simulink model "base_model_2021a_WS2223_controlled"  (R2021a)
settings: Solver=FixedStepDiscrete  StartTime=0.0  StopTime=10  FixedStep=0.01  RelTol=1e-3
libraries: simulink x5, pid_lib x1
settings Model: Creator=paulplusx  LastModifiedBy=erikd
settings SolverCC: AlgebraicLoopSolver=TrustRegion
settings DebuggingCC: SFMachineParentedDataDiag=warning

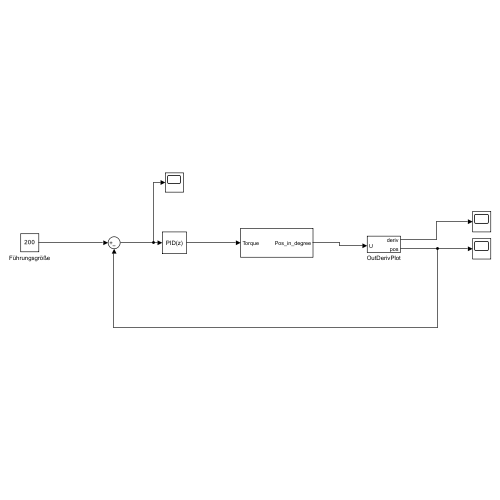
[thumbnail: Simulink's stored preview of the top-level diagram]
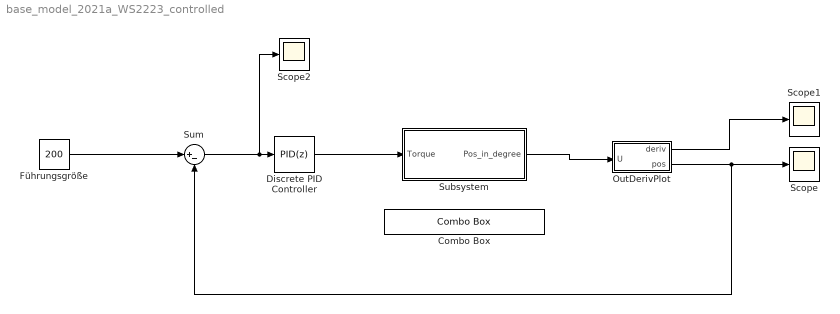
== system base_model_2021a_WS2223_controlled ==
  Combo Box : ComboBox  LabelPosition=Hide  SelectedLabel=ZERO
      settings: Values={{'ZERO', 'TYPE1', 'TYPE2', 'TYPE3', 'TYPE4', 'TYPE5', 'TYPE6', 'TYPE7', 'TYPE8', 'TYPE9'}, [0 1 2 3 4 5 6 7 8 9]}
  Discrete PID Controller : pid_lib/PID Controller  Controller=PID  Form=Parallel  TimeDomain=Discrete-time  UseExternalTs=off  SampleTime=-1  IntegratorMethod=Forward Euler  FilterMethod=Forward Euler  ControllerParametersSource=internal  P=1.02  I=0.236  D=0.059  N=100  UseFilter=on  TunerSelectOption=Transfer Function Based (PID Tuner App)  InitialConditionSource=internal  InitialConditionForIntegrator=0  InitialConditionForFilter=0  DifferentiatorICPrevScaledInput=0  ExternalReset=none  TrackingMode=off  Kt=1  LimitOutput=off  SatLimitsSource=internal  UpperSaturationLimit=inf  LowerSaturationLimit=-inf  LinearizeAsGain=off  AntiWindupMode=none  Kb=1  POutMin=[]  POutMax=[]  IOutMin=[]  IOutMax=[]  DOutMin=[]  DOutMax=[]  NOutMin=[]  NOutMax=[]  SumOutDataTypeStr=int32  SumOutMin=[]  SumOutMax=[]  SaturationOutMin=[]  SaturationOutMax=[]  PParamMin=[]  PParamMax=[]  IParamMin=[]  IParamMax=[]  DParamMin=[]  DParamMax=[]  NParamMin=[]  NParamMax=[]  KbParamMin=[]  KbParamMax=[]  KtParamMin=[]  KtParamMax=[]  KbOutMin=[]  KbOutMax=[]  KtOutMin=[]  KtOutMax=[]  IntegratorOutMin=[]  IntegratorOutMax=[]  FilterOutMin=[]  FilterOutMax=[]  SumI1OutMin=[]  SumI1OutMax=[]  SumI2OutMin=[]  SumI2OutMax=[]  SumI3OutMin=[]  SumI3OutMax=[]  SumI4OutMin=[]  SumI4OutMax=[]  SumDOutMin=[]  SumDOutMax=[]  DifferentiatorOutMin=[]  DifferentiatorOutMax=[]  FilterDiffOutCoefMin=[]  FilterDiffOutCoefMax=[]  ReciprocalOutMin=[]  ReciprocalOutMax=[]  SumDenOutMin=[]  SumDenOutMax=[]  SumNumOutMin=[]  SumNumOutMax=[]  DivideOutMin=[]  DivideOutMax=[]  UdiffTsProdOutMin=[]  UdiffTsProdOutMax=[]  NTsProdOutMin=[]  NTsProdOutMax=[]  UintegralTsProdOutMin=[]  UintegralTsProdOutMax=[]  UngainTsProdOutMin=[]  UngainTsProdOutMax=[]  IntegratorContinuousStateAttributes=''  IntegratorStateMustResolveToSignalObject=off  IntegratorRTWStateStorageClass=Auto  FilterContinuousStateAttributes=''  FilterStateMustResolveToSignalObject=off  FilterRTWStateStorageClass=Auto  ParallelPVariant=InternalParameters  IdealPVariant=Disabled  IVariant=InternalParameters  DVariant=InternalParameters  IntegratorVariant=Discrete  SatVariant=Disabled  AWVariant=Passthrough  PCopyVariant=Disabled  TRVariant=Disabled  FdbkBlocksVariant=Forward  IdealPFdbkVariant=Disabled  SatFdbkVariant=Disabled  DerivativeFilterVariant=ForwardEulerFilter  NVariant=InternalParameters  NCopyVariant=Disabled  FilterICVariant=InternalICsFilter  IntegratorICVariant=InternalICs  ExternalResetVariant=Disabled  TRSumVariant=Passthrough  SumFdbkVariant=Disabled  SumVariant=Sum_PID  TsampFilterVariant=InternalTs  TsampNgainVariant=Passthrough  TsampIntegralVariant=Passthrough  ExternalSaturationOutDataTypeStr=Inherit: Same as second input
  Führungsgröße : Constant  Value=200
  OutDerivPlot : Subsystem
  Scope : Scope
  Scope1 : Scope
  Scope2 : Scope
  Subsystem : Subsystem
  Sum : Sum  Inputs=|+-
  wires:
  Subsystem/1(Pos_in_degree) -> OutDerivPlot/1(U)
  Führungsgröße/1 -> Sum/1
  OutDerivPlot/2(pos) -> Scope/1, Sum/2
  Sum/1 -> Scope2/1, Discrete PID Controller/1
  Discrete PID Controller/1 -> Subsystem/1(Torque)
  OutDerivPlot/1(deriv) -> Scope1/1

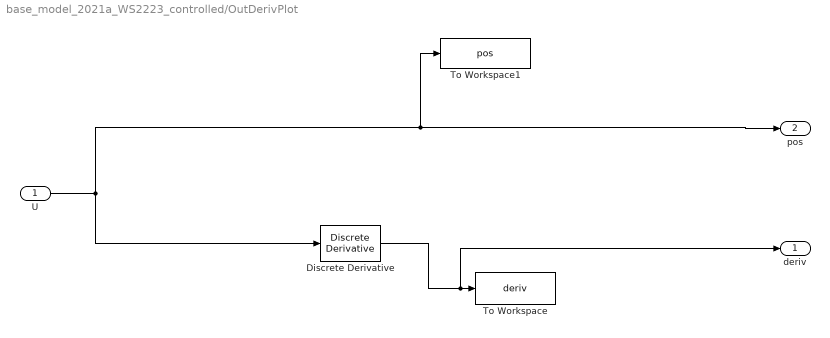
== system base_model_2021a_WS2223_controlled/OutDerivPlot ==
  U : Inport
  Discrete Derivative : simulink/Discrete/Discrete Derivative  gainval=1.0  ICPrevScaledInput=0.0  OutMin=[]  OutMax=[]  OutDataType=fixdt(1, 16)  OutScaling=2^-10  DoSatur=off
  To Workspace : ToWorkspace  VariableName=deriv  SaveFormat=Timeseries  SampleTime=-1
  To Workspace1 : ToWorkspace  VariableName=pos  SaveFormat=Timeseries  SampleTime=-1
  deriv : Outport
  pos : Outport  Port=2
  wires:
  U/1 -> pos/1, To Workspace1/1, Discrete Derivative/1
  Discrete Derivative/1 -> deriv/1, To Workspace/1

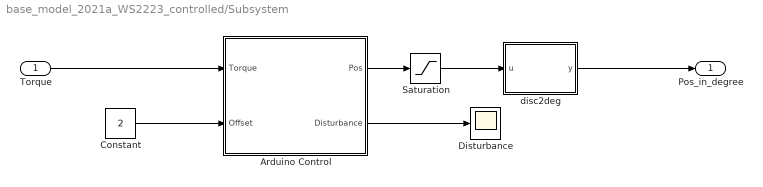
== system base_model_2021a_WS2223_controlled/Subsystem ==
  Torque : Inport
  Arduino Control : Subsystem
  Constant : Constant  Value=2  OutDataTypeStr=int32
  Disturbance : Scope
  Saturation : Saturate  UpperLimit=1024  LowerLimit=0
  disc2deg : MATLAB Function  TreatAsAtomicUnit=on
  Pos_in_degree : Outport
  wires:
  Arduino Control/1(Pos) -> Saturation/1
  Constant/1 -> Arduino Control/2(Offset)
  Arduino Control/2(Disturbance) -> Disturbance/1
  Saturation/1 -> disc2deg/1(u)
  disc2deg/1(y) -> Pos_in_degree/1
  Torque/1 -> Arduino Control/1(Torque)

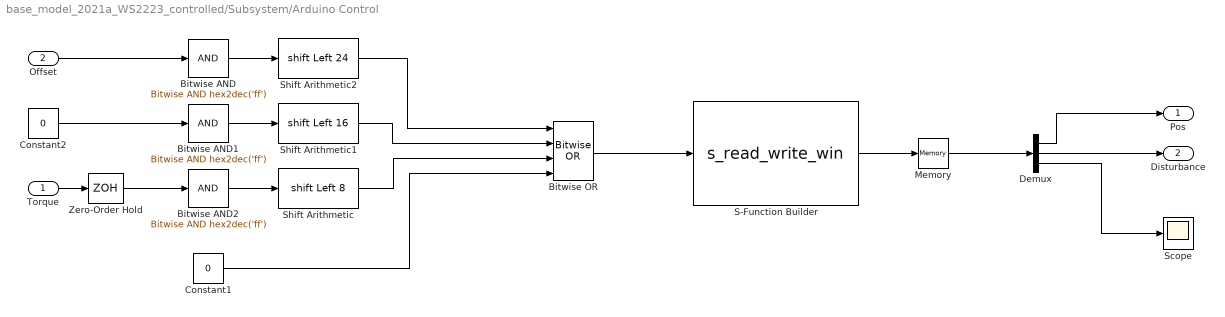
== system base_model_2021a_WS2223_controlled/Subsystem/Arduino Control ==
  Torque : Inport
  Offset : Inport  Port=2
  Bitwise AND : simulink/Logic and Bit Operations/Bitwise Operator  logicop=AND  UseBitMask=on  BitMask=hex2dec('ff')  BitMaskRealWorld=Stored Integer
  Bitwise AND1 : simulink/Logic and Bit Operations/Bitwise Operator  logicop=AND  UseBitMask=on  BitMask=hex2dec('ff')  BitMaskRealWorld=Stored Integer
  Bitwise AND2 : simulink/Logic and Bit Operations/Bitwise Operator  logicop=AND  UseBitMask=on  BitMask=hex2dec('ff')  BitMaskRealWorld=Stored Integer
  Bitwise OR : simulink/Logic and Bit Operations/Bitwise Operator  logicop=OR  UseBitMask=off  NumInputPorts=4  BitMask=bin2dec('11011001')  BitMaskRealWorld=Stored Integer
  Constant1 : Constant  Value=0  OutDataTypeStr=int32  SampleTime=-1
  Constant2 : Constant  Value=0  OutDataTypeStr=int32  SampleTime=-1
  Demux : Demux  Outputs=3
  Memory : Memory
  S-Function Builder : S-Function  FunctionName=s_read_write_win  SFunctionModules=s_read_write_win_wrapper  SFunctionDeploymentMode=off  EnableBusSupport=off  mask(S-Function Builder){}
      mask help: Simulink:masks:SFunctionBuilder_MD
      mask init:
      | val = [[.9  0.75 0.75 1 1 .9 .9 1]',[1 1 0.75 0.75 .9 .9 1 .9]'];try , sys = get_param(gcb,'SfunBuilderFcnName');if isempty(sys), sys = get_param(gcb,'FunctionName'); end,catch, sys = get_param(gcb,'FunctionName'); end
      settings: CopyFcn=set_param(gcbh,'LinkStatus','none')  OpenFcn=sfunctionwizard(gcbh)
      mask Display:
      | plot(val(:,1),val(:,2))
      | disp(sys)
      | port_label('input',1,'TX')
      | port_label('output',1,'RX')
  Scope : Scope
  Shift Arithmetic : ArithShift  BitShiftNumber=8  BitShiftDirection=Left
  Shift Arithmetic1 : ArithShift  BitShiftNumber=16  BitShiftDirection=Left
  Shift Arithmetic2 : ArithShift  BitShiftNumber=24  BitShiftDirection=Left
  Zero-Order Hold : ZeroOrderHold  SampleTime=-1
  Pos : Outport
  Disturbance : Outport  Port=2
  wires:
  Shift Arithmetic2/1 -> Bitwise OR/1
  Zero-Order Hold/1 -> Bitwise AND2/1
  Bitwise AND2/1 -> Shift Arithmetic/1
  Shift Arithmetic1/1 -> Bitwise OR/2
  Bitwise AND/1 -> Shift Arithmetic2/1
  Bitwise OR/1 -> S-Function Builder/1
  Bitwise AND1/1 -> Shift Arithmetic1/1
  Shift Arithmetic/1 -> Bitwise OR/3
  Memory/1 -> Demux/1
  S-Function Builder/1 -> Memory/1
  Constant2/1 -> Bitwise AND1/1
  Offset/1 -> Bitwise AND/1
  Torque/1 -> Zero-Order Hold/1
  Constant1/1 -> Bitwise OR/4
  Demux/1 -> Pos/1
  Demux/2 -> Disturbance/1
  Demux/3 -> Scope/1

== matlab function base_model_2021a_WS2223_controlled/Subsystem/disc2deg ==
  data: u input; y output
function y = fcn(u)

y = mod(360.0/1024.0 * u + 98, 360);
